simulink model "BFSK_MODEM"  (R2024a)
settings: Solver=VariableStepAuto  StartTime=0.0  StopTime=3.5/B  MaxStep=3.5/(B*1000)  MinStep=3/(B*1000)  RelTol=1e-3
undefined symbols (not defined in the file or in its folder): B, f0, f1, f2
libraries: dspsigops x1, simulink x1
settings Model: Creator=pc  LastModifiedBy=pc

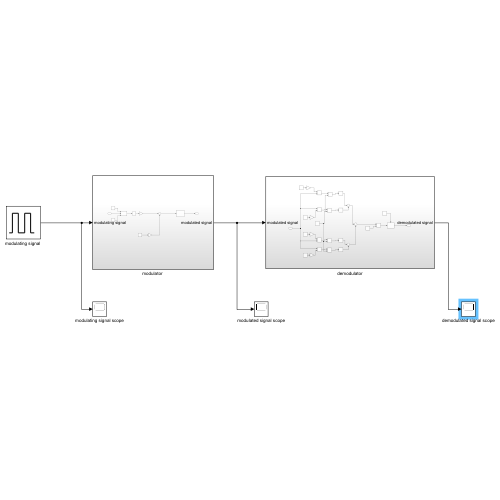
[thumbnail: Simulink's stored preview of the top-level diagram]
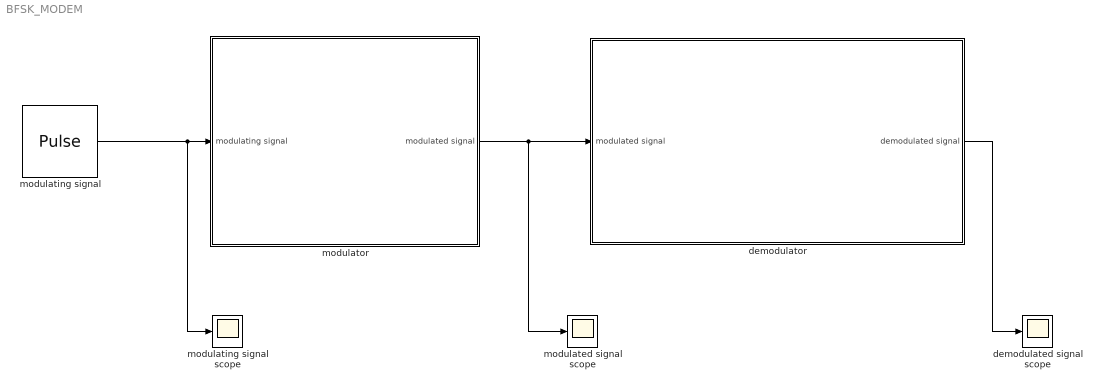
== system BFSK_MODEM ==
  demodulated signal scope : Scope
  demodulator : Subsystem
  modulated signal scope : Scope
  "modulating signal " : DiscretePulseGenerator  PulseType=Time based  Period=2/B  PulseWidth=50
  modulating signal scope : Scope
  "modulator " : Subsystem
  wires:
  "modulator "/1(modulated signal) -> modulated signal scope/1, demodulator/1(modulated signal)
  "modulating signal "/1 -> modulating signal scope/1, "modulator "/1(modulating signal)
  demodulator/1(demodulated signal) -> demodulated signal scope/1

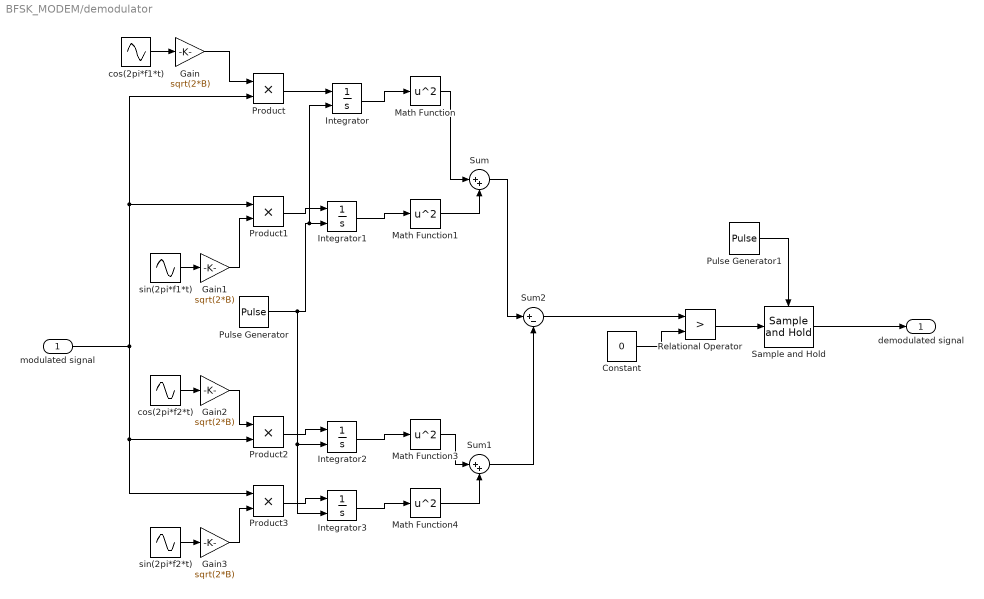
== system BFSK_MODEM/demodulator ==
  modulated signal : Inport
  Constant : Constant  Value=0
  Gain{,1..3} (4 alike) : Gain  Gain=sqrt(2*B)
  Integrator{,1..3} (4 alike) : Integrator  ExternalReset=rising
  Math Function{,1,3..4} (4 alike) : Math  Operator=square
  Product{,1..3} (4 alike) : Product
  Pulse Generator : DiscretePulseGenerator  PulseType=Time based  Period=1/B  PulseWidth=50
  Pulse Generator1 : DiscretePulseGenerator  PulseType=Time based  Period=1/B  PulseWidth=50  PhaseDelay=-10^(-7)
  Relational Operator : RelationalOperator  Operator=>  OutDataTypeStr=boolean  RndMeth=Simplest  InputSameDT=off
  Sample and Hold : dspsigops/Sample and Hold  trig=Rising edge  initCond=0  latchinput=off
  Sum : Sum  Inputs=|++
  Sum1 : Sum  Inputs=|++
  Sum2 : Sum  Inputs=|+-
  cos(2pi*f1*t) : Sin  Frequency=2*pi*f1  Phase=pi/2  SampleTime=0
  cos(2pi*f2*t) : Sin  Frequency=2*pi*f2  Phase=pi/2  SampleTime=0
  sin(2pi*f1*t) : Sin  Frequency=2*pi*f1  SampleTime=0
  sin(2pi*f2*t) : Sin  Frequency=2*pi*f2  SampleTime=0
  demodulated signal : Outport
  wires:
  modulated signal/1 -> Product3/1, Product2/2, Product/2, Product1/1
  Integrator2/1 -> Math Function3/1
  Sum/1 -> Sum2/1
  Math Function4/1 -> Sum1/2
  Math Function/1 -> Sum/1
  Math Function3/1 -> Sum1/1
  Product2/1 -> Integrator2/1
  Integrator3/1 -> Math Function4/1
  Sum1/1 -> Sum2/2
  Product3/1 -> Integrator3/1
  Product/1 -> Integrator/1
  Integrator/1 -> Math Function/1
  Math Function1/1 -> Sum/2
  Integrator1/1 -> Math Function1/1
  Sum2/1 -> Relational Operator/1
  Product1/1 -> Integrator1/1
  Pulse Generator/1 -> Integrator3/2, Integrator2/2, Integrator/2, Integrator1/2
  cos(2pi*f1*t)/1 -> Gain/1
  Gain/1 -> Product/1
  sin(2pi*f1*t)/1 -> Gain1/1
  Gain1/1 -> Product1/2
  cos(2pi*f2*t)/1 -> Gain2/1
  sin(2pi*f2*t)/1 -> Gain3/1
  Gain3/1 -> Product3/2
  Gain2/1 -> Product2/1
  Constant/1 -> Relational Operator/2
  Relational Operator/1 -> Sample and Hold/1
  Sample and Hold/1 -> demodulated signal/1
  Pulse Generator1/1 -> Sample and Hold/Trigger

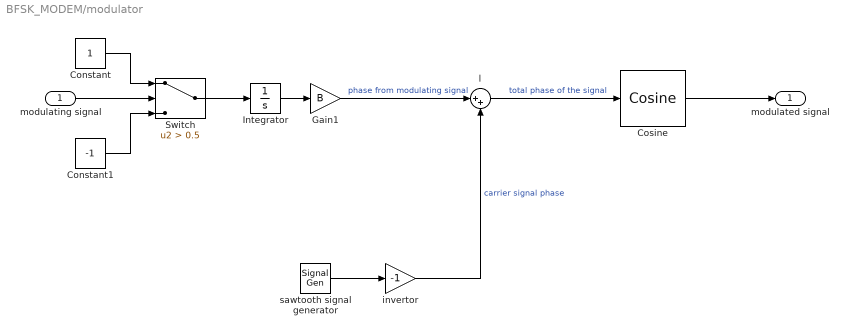
== system BFSK_MODEM/modulator  ==
  modulating signal : Inport
  Constant : Constant
  Constant1 : Constant  Value=-1
  Cosine : simulink/Lookup Tables/Cosine  Formula=cos(2*pi*u)  NumDataPoints=(2^12)+1  OutputWordLength=32  InternalRulePriority=Speed
  Gain1 : Gain  Gain=B
  Integrator : Integrator
  Switch : Switch  Criteria=u2 > Threshold  Threshold=0.5  SaturateOnIntegerOverflow=off  InputSameDT=off
  invertor : Gain  Gain=-1
  l : Sum  Inputs=|++
  sawtooth signal generator : SignalGenerator  WaveForm=sawtooth  Frequency=f0/2
  modulated signal : Outport
  wires:
  Gain1/1 -> l/1  "phase from modulating signal"
  Cosine/1 -> modulated signal/1
  Integrator/1 -> Gain1/1
  invertor/1 -> l/2  "carrier signal phase"
  sawtooth signal generator/1 -> invertor/1
  modulating signal/1 -> Switch/2
  Constant/1 -> Switch/1
  Constant1/1 -> Switch/3
  Switch/1 -> Integrator/1
  l/1 -> Cosine/1  "total phase of the signal"
